simulink model "ulcine"  (R2017a)
settings: Solver=VariableStepAuto  StartTime=0.0  StopTime=10.0  RelTol=1e-3
libraries: simulink x2
settings Model: Creator=Dell  LastModifiedBy=Dell

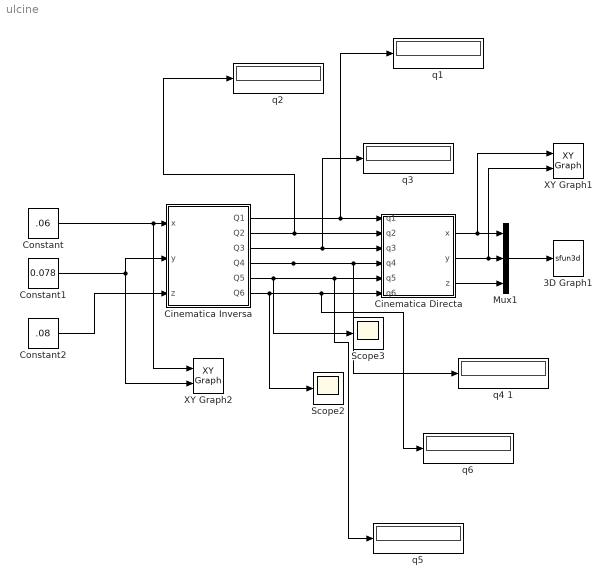
== system ulcine ==
  3D Graph1 : S-Function  LoadFcn=if exist('sfun3d','file'), sfun3d([],[],[],'LoadBlock'); end  FunctionName=sfun3d  Parameters=ax,T,np,cp,gd,ls,mk,mx,hd,tb  SFunctionDeploymentMode=off  EnableBusSupport=off  mask(3D Graph){np=1, ax=[-.5 0.5 -.5 0.5 -.5 .5], mx=2000, T=-1, cp=[370 -234 -207], gd=on, hd=on, tb=off, ls=-, mk=none}
      mask prompts: np "Number of moving points (lines)"; ax "Range: [xmin xmax  ymin ymax zmin zmax]"; mx "Max number of points in each line"; T "Sampling Time"; cp "Camera position (use [0 0 1] for 2D XY view)"; gd "Grid (on|off)"; hd "HeadMarkers (on|off)"; tb "Toolbar (on|off)"; ls "LineStyle"; mk "LineMarker"
      mask help:
      | This block plots the position of several points in the XYZ space. The input contains the coordinates of all the points (x1,y1,z1,x2,y2,z2,...).
      | The number of moving points (lines), the XYZ ranges, sampling time, camera position, and grid (among other things) can be set as mask parameters.
      settings: CopyFcn=if exist('sfun3d','file'), sfun3d([],[],[],'CopyBlock'); end  DeleteFcn=if exist('sfun3d','file'), sfun3d([],[],[],'DeleteBlock'); end  NameChangeFcn=if exist('sfun3d','file'), sfun3d([],[],[],'NameChange'); end
      mask Help:
      | This block plots the position of several points in the XYZ space. The input contains the coordinates of all the points (x1,y1,z1,x2,y2,z2,...).
      | The number of moving points (lines), the XYZ ranges, sampling time, camera position, and grid (among other things) can be set as mask parameters.
      mask TypeOptions ls: - | -- | : | -. | none
      mask TypeOptions mk: none | . | + | o | * | x | square | diamond | v | ^ | > | < | pentagram | hexagram
      mask Display: plot([.05 .95 .95 .05 .05],[.45 .45 .95 .95 .45], 0.5+cos(0:0.1:2*pi)*0.3,0.7+sin(0:0.1:2*pi)*0.2)
  Cinematica Directa : MATLAB Function  TreatAsAtomicUnit=on
  "Cinematica Inversa " : MATLAB Function  TreatAsAtomicUnit=on
  Constant : Constant  Value=.06
  Constant1 : Constant  Value=0.078
  Constant2 : Constant  Value=.08
  Mux1 : Mux  Inputs=3
  Scope2 : Scope
  Scope3 : Scope
  XY Graph1 : simulink/Sinks/XY Graph  xmin=-.5  xmax=.5  ymin=-.5  ymax=.5  st=-1
  XY Graph2 : simulink/Sinks/XY Graph  xmin=-.5  xmax=.5  ymin=-.5  ymax=.5  st=-1
  "q1 " : Display
  "q2 " : Display
  "q3 " : Display
  q4 1 : Display
  "q5 " : Display
  "q6 " : Display
  wires:
  Cinematica Directa/3(z) -> Mux1/3
  Cinematica Directa/2(y) -> XY Graph1/2, Mux1/2
  "Cinematica Inversa "/6(Q6) -> "q6 "/1, Cinematica Directa/6(q6), Scope2/1
  "Cinematica Inversa "/4(Q4) -> q4 1/1, Cinematica Directa/4(q4)
  Constant/1 -> XY Graph2/1, "Cinematica Inversa "/1(x)
  "Cinematica Inversa "/5(Q5) -> "q5 "/1, Cinematica Directa/5(q5), Scope3/1
  Cinematica Directa/1(x) -> XY Graph1/1, Mux1/1
  "Cinematica Inversa "/1(Q1) -> "q1 "/1, Cinematica Directa/1(q1)
  Constant1/1 -> "Cinematica Inversa "/2(y), XY Graph2/2
  Mux1/1 -> 3D Graph1/1
  Constant2/1 -> "Cinematica Inversa "/3(z)
  "Cinematica Inversa "/3(Q3) -> "q3 "/1, Cinematica Directa/3(q3)
  "Cinematica Inversa "/2(Q2) -> "q2 "/1, Cinematica Directa/2(q2)

== matlab function ulcine/Cinematica Directa ==
  data: x output; q1 input; y output; z output; q2 input; q3 input; q4 input; q5 input; q6 input
function [x,y,z]= fcn(q1,q2,q3,q4,q5,q6)
 %segunda CD es de alex                                                                                          
% longitud en metros 
l1=0.190;
l2=.04;
l3=0.110;
l4=0.210;
l5=0.05;

Pos=[l2*cos(q1) + l3*cos(q1)*cos(q2) + l4*cos(q1)*cos(q2)*cos(q3) - l4*cos(q1)*sin(q2)*sin(q3) + l5*sin(q1)*sin(q4)*sin(q5) + l5*cos(q1)*cos(q2)*cos(q3)*cos(q5) - l5*cos(q1)*cos(q5)*sin(q2)*sin(q3) - l5*cos(q1)*cos(q2)*cos(q4)*sin(q3)*sin(q5) - l5*cos(q1)*cos(q3)*cos(q4)*sin(q2)*sin(q5);
    l2*sin(q1) + l3*cos(q2)*sin(q1) + l4*cos(q2)*cos(q3)*sin(q1) - l5*cos(q1)*sin(q4)*sin(q5) - l4*sin(q1)*sin(q2)*sin(q3) + l5*cos(q2)*cos(q3)*cos(q5)*sin(q1) - l5*cos(q5)*sin(q1)*sin(q2)*sin(q3) - l5*cos(q2)*cos(q4)*sin(q1)*sin(q3)*sin(q5) - l5*cos(q3)*cos(q4)*sin(q1)*sin(q2)*sin(q5); 
    l1 + l3*sin(q2) + l4*cos(q2)*sin(q3) + l4*cos(q3)*sin(q2) + l5*cos(q2)*cos(q5)*sin(q3) + l5*cos(q3)*cos(q5)*sin(q2) + l5*cos(q2)*cos(q3)*cos(q4)*sin(q5) - l5*cos(q4)*sin(q2)*sin(q3)*sin(q5)]

%cinemática directa 
%x = Pos(1);
%y = Pos(2); %signo (- )para que cambie el cuadrante 
%z = Pos(3);

x=Pos(1);
y=Pos(2);
z=Pos(3);

== matlab function ulcine/Cinematica Inversa  ==
  data: Q1 output; x input; Q2 output; Q3 output; y input; z input; Q4 output; Q5 output; Q6 output
function [Q1,Q2,Q3,Q4,Q5,Q6] = fcn(x,y,z) % cinematic acon valores nuevos 
l1=0.190;
l2=0.04;
l3=0.110;
l4=0.210;
l5=0.05;


%%%codo Arriba
r=sqrt(x^2+y^2);
ca=r-l2; %%
co=z-l1; %%
Q1 = atan2(y,x);
hi=sqrt(ca^2+co^2);
C3 =((-hi^2+l3^2+l4^2)/(-2*l4*l3));
Q3= atan2(-sqrt(1-C3^2),C3); %%Codo Arriba
Q2=atan2(co,ca)-atan2(l4*sin(Q3),l3+l4*cos(Q3));


Q4=atan2(cos(Q1),sin(Q2+Q3)*sin(Q1))
Q5=atan2(sqrt(1-(cos(Q2+Q3)*cos(Q1))),cos(Q2+Q3)*cos(Q1))
Q6=atan2(sin(Q2+Q3),cos(Q2+Q3)*cos(Q1))
